simulink model "Simulink_Program_DCFC_Normal"  (R2023b)
settings: Solver=VariableStepAuto  StartTime=0.0  StopTime=1  RelTol=1e-3
libraries: fl_lib x12, nesl_utility x10, ee_lib x7
settings Model: Creator=romul  LastModifiedBy=OWNER

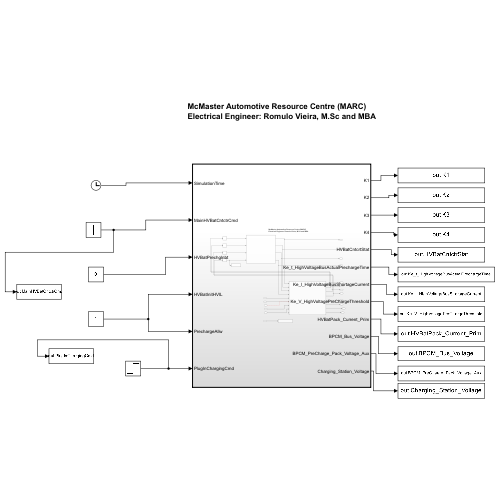
[thumbnail: Simulink's stored preview of the top-level diagram]
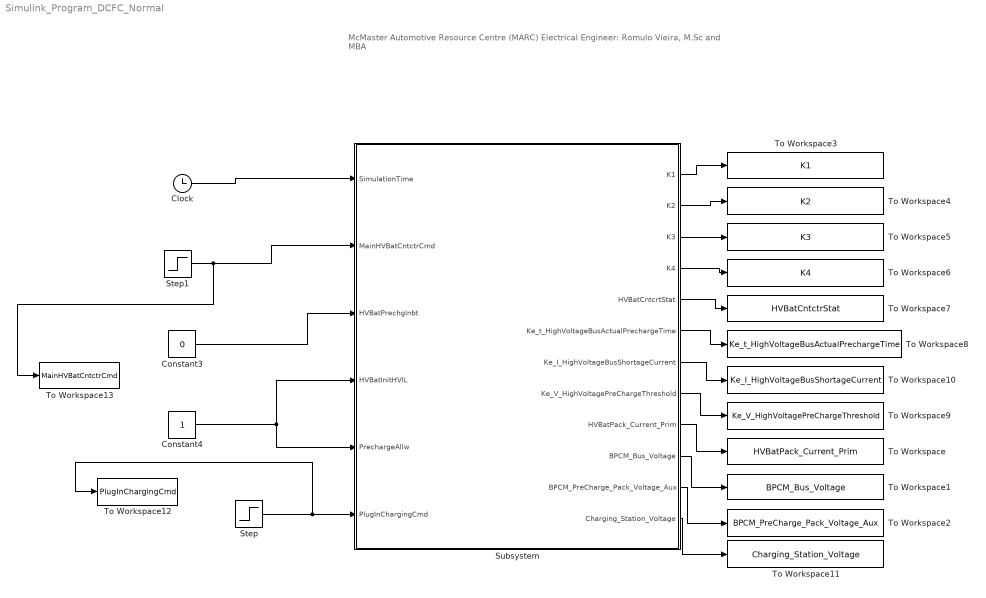
== system Simulink_Program_DCFC_Normal ==
  note: McMaster Automotive Resource Centre (MARC)
      | Electrical Engineer: Romulo Vieira, M.Sc and MBA
  Clock : Clock
  Constant3 : Constant  Value=0
  Constant4 : Constant
  Step : Step  Time=0.5  SampleTime=0.001
  Step1 : Step  Time=0.5  SampleTime=0.001
  Subsystem : Subsystem  TreatAsAtomicUnit=on
  To Workspace : ToWorkspace  VariableName=HVBatPack_Current_Prim  SampleTime=-1
  To Workspace1 : ToWorkspace  VariableName=BPCM_Bus_Voltage  SampleTime=-1
  To Workspace10 : ToWorkspace  VariableName=Ke_I_HighVoltageBusShortageCurrent  SampleTime=-1
  To Workspace11 : ToWorkspace  VariableName=Charging_Station_Voltage  SampleTime=-1
  To Workspace12 : ToWorkspace  VariableName=PlugInChargingCmd  SaveFormat=Timeseries  SampleTime=-1
  To Workspace13 : ToWorkspace  VariableName=MainHVBatCntctrCmd  SaveFormat=Timeseries  SampleTime=-1
  To Workspace2 : ToWorkspace  VariableName=BPCM_PreCharge_Pack_Voltage_Aux  SampleTime=-1
  To Workspace3 : ToWorkspace  VariableName=K1  SampleTime=-1
  To Workspace4 : ToWorkspace  VariableName=K2  SampleTime=-1
  To Workspace5 : ToWorkspace  VariableName=K3  SampleTime=-1
  To Workspace6 : ToWorkspace  VariableName=K4  SampleTime=-1
  To Workspace7 : ToWorkspace  VariableName=HVBatCntctrStat  SampleTime=-1
  To Workspace8 : ToWorkspace  VariableName=Ke_t_HighVoltageBusActualPrechargeTime  SampleTime=-1
  To Workspace9 : ToWorkspace  VariableName=Ke_V_HighVoltagePreChargeThreshold  SampleTime=-1
  wires:
  Subsystem/1(K1) -> To Workspace3/1
  Subsystem/2(K2) -> To Workspace4/1
  Subsystem/3(K3) -> To Workspace5/1
  Subsystem/4(K4) -> To Workspace6/1
  Subsystem/5(HVBatCntcrtStat) -> To Workspace7/1
  Subsystem/6(Ke_t_HighVoltageBusActualPrechargeTime) -> To Workspace8/1
  Subsystem/7(Ke_I_HighVoltageBusShortageCurrent) -> To Workspace10/1
  Clock/1 -> Subsystem/1(SimulationTime)
  Step1/1 -> To Workspace13/1, Subsystem/2(MainHVBatCntctrCmd)
  Constant3/1 -> Subsystem/3(HVBatPrechgInbt)
  Constant4/1 -> Subsystem/5(PrechargeAllw), Subsystem/4(HVBatInitHVIL)
  Subsystem/10(BPCM_Bus_Voltage) -> To Workspace1/1
  Subsystem/9(HVBatPack_Current_Prim) -> To Workspace/1
  Subsystem/11(BPCM_PreCharge_Pack_Voltage_Aux) -> To Workspace2/1
  Subsystem/8(Ke_V_HighVoltagePreChargeThreshold) -> To Workspace9/1
  Subsystem/12(Charging_Station_Voltage) -> To Workspace11/1
  Step/1 -> To Workspace12/1, Subsystem/6(PlugInChargingCmd)

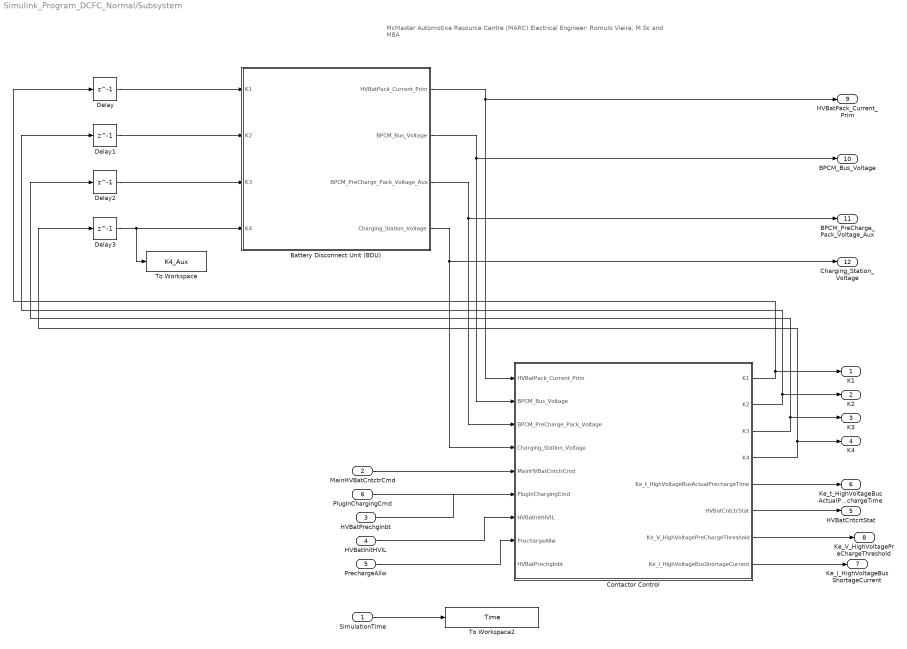
== system Simulink_Program_DCFC_Normal/Subsystem ==
  note: McMaster Automotive Resource Centre (MARC)
      | Electrical Engineer: Romulo Vieira, M.Sc and MBA
  SimulationTime : Inport
  MainHVBatCntctrCmd : Inport  Port=2
  HVBatPrechgInbt : Inport  Port=3
  HVBatInitHVIL : Inport  Port=4
  PrechargeAllw : Inport  Port=5
  PlugInChargingCmd : Inport  Port=6
  Battery Disconnect Unit (BDU) : Subsystem  TreatAsAtomicUnit=on
  Contactor Control : Subsystem  TreatAsAtomicUnit=on  SystemSampleTime=0.001
  Delay{,1..3} (4 alike) : Delay  DelayLength=1
  To Workspace : ToWorkspace  VariableName=K4_Aux  SaveFormat=Timeseries  SampleTime=-1
  To Workspace2 : ToWorkspace  VariableName=Time  SampleTime=0.001
  K1 : Outport
  K2 : Outport  Port=2
  K3 : Outport  Port=3
  K4 : Outport  Port=4
  HVBatCntcrtStat : Outport  Port=5
  Ke_t_HighVoltageBusActualPrechargeTime : Outport  Port=6
  Ke_I_HighVoltageBusShortageCurrent : Outport  Port=7
  Ke_V_HighVoltagePreChargeThreshold : Outport  Port=8
  HVBatPack_Current_Prim : Outport  Port=9
  BPCM_Bus_Voltage : Outport  Port=10
  BPCM_PreCharge_Pack_Voltage_Aux : Outport  Port=11
  Charging_Station_Voltage : Outport  Port=12
  wires:
  Battery Disconnect Unit (BDU)/1(HVBatPack_Current_Prim) -> Contactor Control/1(HVBatPack_Current_Prim), HVBatPack_Current_Prim/1
  Battery Disconnect Unit (BDU)/2(BPCM_Bus_Voltage) -> Contactor Control/2(BPCM_Bus_Voltage), BPCM_Bus_Voltage/1
  MainHVBatCntctrCmd/1 -> Contactor Control/5(MainHVBatCntctrCmd)
  HVBatPrechgInbt/1 -> ?
  HVBatInitHVIL/1 -> Contactor Control/7(HVBatInitHVIL)
  PrechargeAllw/1 -> Contactor Control/8(PrechargeAllw)
  Contactor Control/1(K1) -> K1/1, Delay/1
  Contactor Control/2(K2) -> K2/1, Delay1/1
  Contactor Control/3(K3) -> K3/1, Delay2/1
  Contactor Control/4(K4) -> K4/1, Delay3/1
  Contactor Control/6(HVBatCntctrStat) -> HVBatCntcrtStat/1
  Contactor Control/5(Ke_t_HighVoltageBusActualPrechargeTime) -> Ke_t_HighVoltageBusActualPrechargeTime/1
  Contactor Control/8(Ke_I_HighVoltageBusShortageCurrent) -> Ke_I_HighVoltageBusShortageCurrent/1
  Contactor Control/7(Ke_V_HighVoltagePreChargeThreshold) -> Ke_V_HighVoltagePreChargeThreshold/1
  Battery Disconnect Unit (BDU)/3(BPCM_PreCharge_Pack_Voltage_Aux) -> BPCM_PreCharge_Pack_Voltage_Aux/1, Contactor Control/3(BPCM_PreCharge_Pack_Voltage)
  Delay/1 -> Battery Disconnect Unit (BDU)/1(K1)
  Delay1/1 -> Battery Disconnect Unit (BDU)/2(K2)
  Delay2/1 -> Battery Disconnect Unit (BDU)/3(K3)
  Delay3/1 -> To Workspace/1, Battery Disconnect Unit (BDU)/4(K4)
  SimulationTime/1 -> To Workspace2/1
  Battery Disconnect Unit (BDU)/4(Charging_Station_Voltage) -> Charging_Station_Voltage/1, Contactor Control/4(Charging_Station_Voltage)
  PlugInChargingCmd/1 -> Contactor Control/6(PlugInChargingCmd)

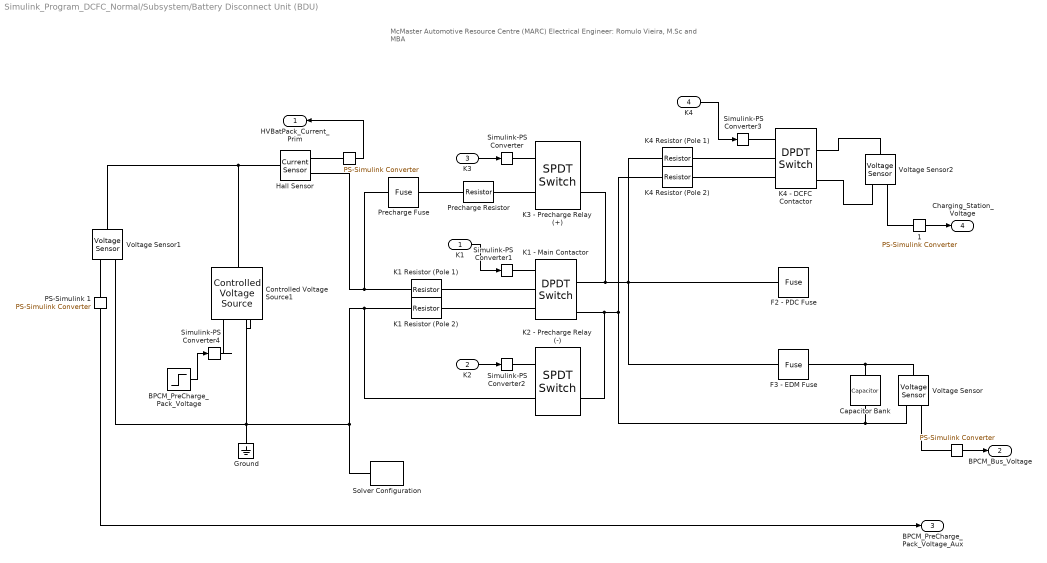
== system Simulink_Program_DCFC_Normal/Subsystem/Battery Disconnect Unit (BDU) ==
  note: McMaster Automotive Resource Centre (MARC)
      | Electrical Engineer: Romulo Vieira, M.Sc and MBA
  K1 : Inport
  K2 : Inport  Port=2
  K3 : Inport  Port=3
  K4 : Inport  Port=4
  "   " : nesl_utility/PS-Simulink Converter  PhysicalDomain=network_engine_domain  SubClassName=ps_output  LeftPortType=input  RightPortType=output  PseudoPeriodic=off  Frequencies=[]  VectorFormat=inherit  Unit=inherit  AffineConversion=off
  " " : nesl_utility/PS-Simulink Converter  PhysicalDomain=network_engine_domain  SubClassName=ps_output  LeftPortType=input  RightPortType=output  PseudoPeriodic=off  Frequencies=[]  VectorFormat=inherit  Unit=inherit  AffineConversion=off
  " 1" : nesl_utility/PS-Simulink Converter  PhysicalDomain=network_engine_domain  SubClassName=ps_output  LeftPortType=input  RightPortType=output  PseudoPeriodic=off  Frequencies=[]  VectorFormat=inherit  Unit=inherit  AffineConversion=off
  BPCM_PreCharge_Pack_Voltage : Step  Time=0  After=450  SampleTime=0.001
  Capacitor Bank : fl_lib/Electrical/Electrical Elements/Capacitor  c=750e-6 F  r=1e-6 Ohm  g=0 1/Ohm  i_specify=off  i_priority=None  i=0 A  i_nominal_specify=off  i_nominal_unit=A  i_nominal_value=1  v_specify=off  v_priority=None  v=0 V  v_nominal_specify=off  v_nominal_unit=V  v_nominal_value=1  vc_specify=on  vc_priority=High  vc=0 V  vc_nominal_specify=off  vc_nominal_unit=V  vc_nominal_value=1
  Controlled Voltage Source1 : fl_lib/Electrical/Electrical Sources/Controlled Voltage Source
  F2 - PDC Fuse : ee_lib/Switches & Breakers/Fuse  prm=1  I_rated=125 A  melt_margin=1  T_fuse=0 s  I2t=1 A^2*s  I_vec=[1.9, 2, 2.5, 30] A  t_vec=[10000, 1, .3, .001] s  R_closed=0.01 Ohm  G_open=1e-8 1/Ohm  exposemeasurement=ee.enum.exposemeasurement.hidden
      settings: InternalSimscapePortConfiguration="{\"Bottom\":[],\"Left\":[{\"id\":\"p\",\"label\":\"\",\"type\":\"foundation.electrical.electrical\"}],\"Right\":[{\"id\":\"n\",\"label\":\"\",\"type\":\"foundation.electrical.electrical\"}],\"Top\":[]}"
  F3 - EDM Fuse : ee_lib/Switches & Breakers/Fuse  prm=1  I_rated=600 A  melt_margin=1  T_fuse=0 s  I2t=1 A^2*s  I_vec=[1.9, 2, 2.5, 30] A  t_vec=[10000, 1, .3, .001] s  R_closed=0.01 Ohm  G_open=1e-8 1/Ohm  exposemeasurement=ee.enum.exposemeasurement.hidden
      settings: InternalSimscapePortConfiguration="{\"Bottom\":[],\"Left\":[{\"id\":\"p\",\"label\":\"\",\"type\":\"foundation.electrical.electrical\"}],\"Right\":[{\"id\":\"n\",\"label\":\"\",\"type\":\"foundation.electrical.electrical\"}],\"Top\":[]}"
  Ground : fl_lib/Electrical/Electrical Elements/Electrical Reference
  Hall Sensor : fl_lib/Electrical/Electrical Sensors/Current Sensor
  K1 - Main Contactor : ee_lib/Switches & Breakers/DPDT Switch  R_closed=0.01 Ohm  G_open=1e-6 S  Threshold=0.5 V  Width=0 V  model_dynamics=0  t_on=1e-3 s  t_off=1e-3 s  initial_vT=0 V
      settings: InternalSimscapePortConfiguration="{\"Bottom\":[],\"Left\":[{\"id\":\"vT\",\"label\":\"vT\",\"type\":\"input\"},{\"id\":\"p1\",\"label\":\"\",\"type\":\"foundation.electrical.electrical\"},{\"id\":\"p2\",\"label\":\"\",\"type\":\"foundation.electrical.electrical\"}],\"Right\":[{\"id\":\"n11\",\"label\":\"\",\"type\":\"foundation.electrical.electrical\"},{\"id\":\"n12\",\"label\":\"\",\"type\":\"foundation.electrical.electrical\"},{\"id\":\"n21\",\"label\":\"\",\"type\":\"foundation.electrical.electrical\"},{\"id\":\"n22\",\"label\":\"\",\"type\":\"foundation.electrical.electrical\"}],\"Top\":[]}"
  K1 Resistor (Pole 1) : fl_lib/Electrical/Electrical Elements/Resistor  R=0.0003 Ohm  i_specify=off  i_priority=None  i=0 A  i_nominal_specify=off  i_nominal_unit=A  i_nominal_value=1  v_specify=off  v_priority=None  v=0 V  v_nominal_specify=off  v_nominal_unit=V  v_nominal_value=1
  K1 Resistor (Pole 2) : fl_lib/Electrical/Electrical Elements/Resistor  R=0.0003 Ohm  i_specify=off  i_priority=None  i=0 A  i_nominal_specify=off  i_nominal_unit=A  i_nominal_value=1  v_specify=off  v_priority=None  v=0 V  v_nominal_specify=off  v_nominal_unit=V  v_nominal_value=1
  K2 - Precharge Relay (-) : ee_lib/Switches & Breakers/SPDT Switch  R_closed=0.01 Ohm  G_open=1e-6 S  Threshold=0.5 V  Width=0 V  model_dynamics=0  t_on=1e-3 s  t_off=1e-3 s  initial_vT=0 V
  K3 - Precharge Relay (+) : ee_lib/Switches & Breakers/SPDT Switch  R_closed=0.01 Ohm  G_open=1e-6 S  Threshold=0.5 V  Width=0 V  model_dynamics=0  t_on=1e-3 s  t_off=1e-3 s  initial_vT=0 V
  K4 - DCFC Contactor : ee_lib/Switches & Breakers/DPDT Switch  R_closed=0.01 Ohm  G_open=1e-6 S  Threshold=0.5 V  Width=0 V  model_dynamics=0  t_on=1e-3 s  t_off=1e-3 s  initial_vT=0 V
      settings: InternalSimscapePortConfiguration="{\"Bottom\":[],\"Left\":[{\"id\":\"vT\",\"label\":\"vT\",\"type\":\"input\"},{\"id\":\"p1\",\"label\":\"\",\"type\":\"foundation.electrical.electrical\"},{\"id\":\"p2\",\"label\":\"\",\"type\":\"foundation.electrical.electrical\"}],\"Right\":[{\"id\":\"n11\",\"label\":\"\",\"type\":\"foundation.electrical.electrical\"},{\"id\":\"n12\",\"label\":\"\",\"type\":\"foundation.electrical.electrical\"},{\"id\":\"n21\",\"label\":\"\",\"type\":\"foundation.electrical.electrical\"},{\"id\":\"n22\",\"label\":\"\",\"type\":\"foundation.electrical.electrical\"}],\"Top\":[]}"
  K4 Resistor (Pole 1) : fl_lib/Electrical/Electrical Elements/Resistor  R=0.0003 Ohm  i_specify=off  i_priority=None  i=0 A  i_nominal_specify=off  i_nominal_unit=A  i_nominal_value=1  v_specify=off  v_priority=None  v=0 V  v_nominal_specify=off  v_nominal_unit=V  v_nominal_value=1
  K4 Resistor (Pole 2) : fl_lib/Electrical/Electrical Elements/Resistor  R=0.0003 Ohm  i_specify=off  i_priority=None  i=0 A  i_nominal_specify=off  i_nominal_unit=A  i_nominal_value=1  v_specify=off  v_priority=None  v=0 V  v_nominal_specify=off  v_nominal_unit=V  v_nominal_value=1
  PS-Simulink 1 : nesl_utility/PS-Simulink Converter  PhysicalDomain=network_engine_domain  SubClassName=ps_output  LeftPortType=input  RightPortType=output  PseudoPeriodic=off  Frequencies=[]  VectorFormat=inherit  Unit=inherit  AffineConversion=off
  Precharge Fuse : ee_lib/Switches & Breakers/Fuse  prm=1  I_rated=600 A  melt_margin=1  T_fuse=0 s  I2t=1 A^2*s  I_vec=[1.9, 2, 2.5, 30] A  t_vec=[10000, 1, .3, .001] s  R_closed=0.01 Ohm  G_open=1e-8 1/Ohm  exposemeasurement=ee.enum.exposemeasurement.hidden
      settings: InternalSimscapePortConfiguration="{\"Bottom\":[],\"Left\":[{\"id\":\"p\",\"label\":\"\",\"type\":\"foundation.electrical.electrical\"}],\"Right\":[{\"id\":\"n\",\"label\":\"\",\"type\":\"foundation.electrical.electrical\"}],\"Top\":[]}"
  Precharge Resistor : fl_lib/Electrical/Electrical Elements/Resistor  R=25 Ohm  i_specify=off  i_priority=None  i=0 A  i_nominal_specify=off  i_nominal_unit=A  i_nominal_value=1  v_specify=off  v_priority=None  v=0 V  v_nominal_specify=off  v_nominal_unit=V  v_nominal_value=1
  Simulink-PS Converter{,1..3} (4 alike) : nesl_utility/Simulink-PS Converter  PhysicalDomain=network_engine_domain  SubClassName=ps_input  LeftPortType=input  RightPortType=output  PseudoPeriodic=off  Frequencies=[]  NoiseDistribution=none  NoiseParameters=[]  Unit=1  AffineConversion=off  FilteringAndDerivatives=provide  SimscapeFilterOrder=1  InputFilterTimeConstant=0.001  UdotUserProvided=0
  Simulink-PS Converter4 : nesl_utility/Simulink-PS Converter  PhysicalDomain=network_engine_domain  SubClassName=ps_input  LeftPortType=input  RightPortType=output  PseudoPeriodic=off  Frequencies=[]  NoiseDistribution=none  NoiseParameters=[]  Unit=1  AffineConversion=off  FilteringAndDerivatives=filter  SimscapeFilterOrder=1  InputFilterTimeConstant=0.0000001  UdotUserProvided=0
  Solver Configuration : nesl_utility/Solver Configuration  PhysicalDomain=network_engine_domain  SubClassName=solver  LeftPortType=input  RightPortType=generic  Tones=[]  Harmonics=[]  SimulateNoise=off  Profile=off  UseLocalSampling=off  EnableSwitchedLinearOptims=on  FrequencyDomain=off  UseCCode=off  RelTol=0.001  AbsTol=0.001  MinStep=1e-09  ToWorkspace=off  RevertToSquareIcSolve=off  NumHomotopyIterations=100  PhasorMode=off  PhasorModeNumHarmonics=1  ConsistencySolver=NEWTON_XTOL_AFTER_FTOL  IndexReductionMethod=DerivativeReplacement  DoDC=off  ResidualTolerance=1e-09  ConsistencyTolSource=GLOBAL  ConsistencyAbsTol=0.001  ConsistencyRelTol=0.001  ConsistencyTolFactor=0.001  UseLocalSolver=off  LocalSolverChoice=NE_BACKWARD_EULER_ADVANCER  ResolveIndetEquations=on  FunctionEvalNumThread=1  LocalSolverSampleTime=0.001  DoFixedCost=off  MaxNonlinIter=3  MaxModeIter=2  ComputeImpulses=off  ImpulseIterations=2  LinearAlgebra=auto  LinearAlgebraNumThread=0  EquationFormulation=NE_TIME_EF  DelaysMemoryBudget=1024  AutomaticFiltering=on  FilteringTimeConstant=0.001  PartitionStorageMethod=AS_NEEDED  PartitionMemoryBudget=1024  PartitionMethod=ROBUST  MultibodyUseLocalSolver=off  MultibodyLocalSolverChoice=ODE1  MultibodyLocalSolverSampleTime=0.001
  Voltage Sensor : fl_lib/Electrical/Electrical Sensors/Voltage Sensor
  Voltage Sensor1 : fl_lib/Electrical/Electrical Sensors/Voltage Sensor
  Voltage Sensor2 : fl_lib/Electrical/Electrical Sensors/Voltage Sensor
  HVBatPack_Current_Prim : Outport
  BPCM_Bus_Voltage : Outport  Port=2
  BPCM_PreCharge_Pack_Voltage_Aux : Outport  Port=3
  Charging_Station_Voltage : Outport  Port=4
  wires:
  K4/1 -> Simulink-PS Converter3/1
  K3/1 -> Simulink-PS Converter/1
  "   "/1 -> HVBatPack_Current_Prim/1
  K1/1 -> Simulink-PS Converter1/1
  K2/1 -> Simulink-PS Converter2/1
  BPCM_PreCharge_Pack_Voltage/1 -> Simulink-PS Converter4/1
  " "/1 -> BPCM_Bus_Voltage/1
  PS-Simulink 1/1 -> BPCM_PreCharge_Pack_Voltage_Aux/1
  " 1"/1 -> Charging_Station_Voltage/1
  connections:
  K1 Resistor (Pole 2)/LConn1 -- K1 - Main Contactor/LConn3
  Capacitor Bank/LConn1 -- Voltage Sensor/LConn1 -- F3 - EDM Fuse/LConn1
  K2 - Precharge Relay (-)/RConn2 -- K1 - Main Contactor/RConn4 -- Voltage Sensor/RConn2 -- Capacitor Bank/RConn1 -- K4 Resistor (Pole 2)/RConn1
  Hall Sensor/RConn2 -- Precharge Fuse/LConn1 -- K1 Resistor (Pole 1)/RConn1
  K3 - Precharge Relay (+)/RConn2 -- K4 Resistor (Pole 1)/RConn1 -- F2 - PDC Fuse/RConn1 -- F3 - EDM Fuse/RConn1 -- K1 - Main Contactor/RConn2
  Precharge Resistor/LConn1 -- K3 - Precharge Relay (+)/LConn2
  Simulink-PS Converter2/RConn1 -- K2 - Precharge Relay (-)/LConn1
  Precharge Resistor/RConn1 -- Precharge Fuse/RConn1
  Simulink-PS Converter1/RConn1 -- K1 - Main Contactor/LConn1
  Controlled Voltage Source1/LConn1 -- Hall Sensor/LConn1 -- Voltage Sensor1/LConn1
  Simulink-PS Converter/RConn1 -- K3 - Precharge Relay (+)/LConn1
  Voltage Sensor/RConn1 -- " "/LConn1
  K4 - DCFC Contactor/LConn1 -- Simulink-PS Converter3/RConn1
  "   "/LConn1 -- Hall Sensor/RConn1
  Simulink-PS Converter4/RConn1 -- Controlled Voltage Source1/RConn1
  Voltage Sensor1/RConn1 -- PS-Simulink 1/LConn1
  K1 Resistor (Pole 1)/LConn1 -- K1 - Main Contactor/LConn2
  Solver Configuration/RConn1 -- Ground/LConn1 -- Voltage Sensor1/RConn2 -- Controlled Voltage Source1/RConn2 -- K2 - Precharge Relay (-)/LConn2 -- K1 Resistor (Pole 2)/RConn1
  K4 - DCFC Contactor/LConn2 -- K4 Resistor (Pole 1)/LConn1
  K4 Resistor (Pole 2)/LConn1 -- K4 - DCFC Contactor/LConn3
  K4 - DCFC Contactor/RConn2 -- Voltage Sensor2/LConn1
  K4 - DCFC Contactor/RConn4 -- Voltage Sensor2/RConn2
  " 1"/LConn1 -- Voltage Sensor2/RConn1

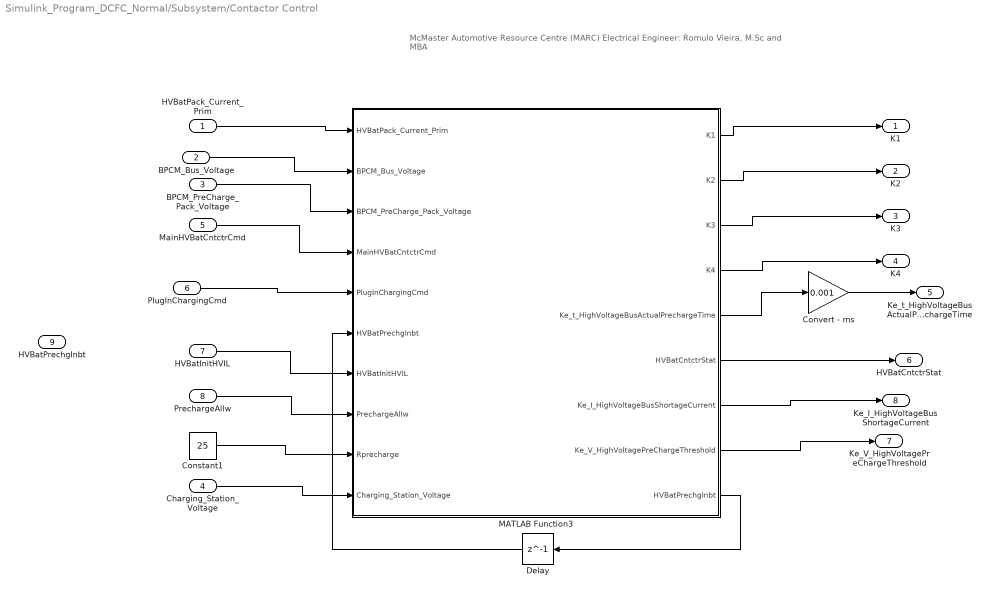
== system Simulink_Program_DCFC_Normal/Subsystem/Contactor Control ==
  note: McMaster Automotive Resource Centre (MARC)
      | Electrical Engineer: Romulo Vieira, M.Sc and MBA
  HVBatPack_Current_Prim : Inport
  BPCM_Bus_Voltage : Inport  Port=2
  BPCM_PreCharge_Pack_Voltage : Inport  Port=3
  Charging_Station_Voltage : Inport  Port=4
  MainHVBatCntctrCmd : Inport  Port=5
  PlugInChargingCmd : Inport  Port=6
  HVBatInitHVIL : Inport  Port=7
  PrechargeAllw : Inport  Port=8
  HVBatPrechgInbt : Inport  Port=9
  Constant1 : Constant  Value=25
  Convert - ms : Gain  Gain=0.001
  Delay : Delay  DelayLength=1
  MATLAB Function3 : MATLAB Function  SystemSampleTime=0.001
  K1 : Outport
  K2 : Outport  Port=2
  K3 : Outport  Port=3
  K4 : Outport  Port=4
  Ke_t_HighVoltageBusActualPrechargeTime : Outport  Port=5
  HVBatCntctrStat : Outport  Port=6
  Ke_V_HighVoltagePreChargeThreshold : Outport  Port=7
  Ke_I_HighVoltageBusShortageCurrent : Outport  Port=8
  wires:
  Constant1/1 -> MATLAB Function3/9(Rprecharge)
  HVBatInitHVIL/1 -> MATLAB Function3/7(HVBatInitHVIL)
  MainHVBatCntctrCmd/1 -> MATLAB Function3/4(MainHVBatCntctrCmd)
  HVBatPack_Current_Prim/1 -> MATLAB Function3/1(HVBatPack_Current_Prim)
  PrechargeAllw/1 -> MATLAB Function3/8(PrechargeAllw)
  MATLAB Function3/1(K1) -> K1/1
  BPCM_PreCharge_Pack_Voltage/1 -> MATLAB Function3/3(BPCM_PreCharge_Pack_Voltage)
  Charging_Station_Voltage/1 -> MATLAB Function3/10(Charging_Station_Voltage)
  MATLAB Function3/2(K2) -> K2/1
  MATLAB Function3/3(K3) -> K3/1
  MATLAB Function3/4(K4) -> K4/1
  MATLAB Function3/6(HVBatCntctrStat) -> HVBatCntctrStat/1
  MATLAB Function3/7(Ke_I_HighVoltageBusShortageCurrent) -> Ke_I_HighVoltageBusShortageCurrent/1
  MATLAB Function3/9(HVBatPrechgInbt) -> Delay/1
  Delay/1 -> MATLAB Function3/6("HVBatPrechgInbt ")
  BPCM_Bus_Voltage/1 -> MATLAB Function3/2(BPCM_Bus_Voltage)
  MATLAB Function3/8(Ke_V_HighVoltagePreChargeThreshold) -> Ke_V_HighVoltagePreChargeThreshold/1
  Convert - ms/1 -> Ke_t_HighVoltageBusActualPrechargeTime/1
  MATLAB Function3/5(Ke_t_HighVoltageBusActualPrechargeTime) -> Convert - ms/1
  PlugInChargingCmd/1 -> MATLAB Function3/5(PlugInChargingCmd)

== matlab function Simulink_Program_DCFC_Normal/Subsystem/Contactor Control/MATLAB Function3 ==
  data: HVBatPack_Current_Prim input; BPCM_Bus_Voltage input; BPCM_PreCharge_Pack_Voltage input; MainHVBatCntctrCmd input; PlugInChargingCmd input; K1 output; HVBatPrechgInbt input; HVBatInitHVIL input; PrechargeAllw input; K2 output; K3 output; K4 output; Ke_t_HighVoltageBusActualPrechargeTime output; HVBatCntctrStat output; Ke_I_HighVoltageBusShortageCurrent output; Ke_V_HighVoltagePreChargeThreshold output; Rprecharge input; HVBatPrechgInbt output; Charging_Station_Voltage input
function [K1, K2, K3, K4, Ke_t_HighVoltageBusActualPrechargeTime, HVBatCntctrStat, Ke_I_HighVoltageBusShortageCurrent, Ke_V_HighVoltagePreChargeThreshold, HVBatPrechgInbt] = ...
    prechargeSequencerNoClock(HVBatPack_Current_Prim, BPCM_Bus_Voltage, ...
    BPCM_PreCharge_Pack_Voltage, MainHVBatCntctrCmd, PlugInChargingCmd, HVBatPrechgInbt, HVBatInitHVIL, PrechargeAllw, Rprecharge, Charging_Station_Voltage)

%-----------------------------------------------------------
% McMaster Automotive Resource Centre (MARC)
% Electrical Engineer: Romulo Vieira, M.Sc and MBA - PhD Candidate
%-----------------------------------------------------------
% Purpose: Manage precharge relay and contactor sequence with retry + inhibit logic
%-----------------------------------------------------------

% HVBatCntctrStat Mapping:
% 0 – Idle/Waiting
% 1 – Precharge Active
% 2 – Precharge Complete (Main contactors closed)
% 3 - DCFC Charging
% 4 – Precharge Failed
% 5 – Inhibit State (cooldown after failure)
% 6 – Contactor Control Shorted (high or low)
% 7 - SNA (Signal Not Available)

% --- Constants ---
Unset_VbusTargetHitIdx             = -1;   % Flag indicating Vbus threshold not yet hit
Min_Samples                        = 0;    % Minimum number of samples where relays and contactor are both active

% Internal Configuration Parameters
Ke_t_PrechargeFailCoolTime             = 3000;   % Cooldown time after one single failed attempt [ms]
Ke_t_ExtraPrechargeFailCoolPenaltyTime = 2000;   % Additional cooldown after two multiple failures [ms]
Ke_t_PrechargeFailMaxPenalty           = 10000;  % Maximum time threshold before enabling precharge inhibit state
Ke_t_BPCM_Precharge_Fail_Penalty_Time  = 15000;  % Hard inhibit time if failures persist [ms]
Ke_I_HighVoltageBusShortageCurrentMin  = 10.8;   % Minimum expected precharge current [A]
Ke_V_HighVoltagePreChargeThreshold     = 0.993 * BPCM_PreCharge_Pack_Voltage;  % Target voltage threshold
Ke_t_HighVoltageBusPrechargeTime  = 100;    % Maximum allowable time for precharging [ms]

% --- Persistent Variables ---
persistent I_buffer idx HVBatCntctrStat_Aux VbusTargetHitIdx ...
    t_counter last_PrechargeAllw Prchrgpnltytimer PrechargeFailCount

if isempty(I_buffer)
    I_buffer               = zeros(Ke_t_HighVoltageBusPrechargeTime,1);
    idx                    = 1;
    HVBatCntctrStat_Aux    = 0;
    VbusTargetHitIdx       = Unset_VbusTargetHitIdx;
    t_counter              = 0;
    last_PrechargeAllw     = 0;
    Prchrgpnltytimer       = 0;
    PrechargeFailCount     = 0; % Represented by k_fail in the flowchart
end

% --- Default Outputs ---
K1 = 0; K2 = 0; K3 = 0; K4 = 0;
HVBatCntctrStat = HVBatCntctrStat_Aux;
Ke_t_HighVoltageBusActualPrechargeTime = 0;
Ke_I_HighVoltageBusShortageCurrent = 0;

% --- Immediate cooldown/inhibit override ---
if Prchrgpnltytimer > 0 && HVBatCntctrStat_Aux ~= 5
    HVBatCntctrStat_Aux = 5;
end

% --- State Machine ---
switch HVBatCntctrStat_Aux
    case 0 % OPEN STATE
        % Set the Battery Contactor States
        K1 = 0; K2 = 0; K3 = 0; K4 = 0;
        % Check Initial conditions
        if PlugInChargingCmd == 1 && MainHVBatCntctrCmd == 1 && HVBatPrechgInbt == 0 && HVBatInitHVIL == 1 && PrechargeAllw == 1
            HVBatCntctrStat_Aux = 3; % DCFC CHARGING
        end
        if PlugInChargingCmd == 0 && MainHVBatCntctrCmd == 1 && HVBatPrechgInbt == 0 && HVBatInitHVIL == 1  && PrechargeAllw == 1
            I_buffer(:) = 0;
            idx = 1;
            VbusTargetHitIdx = Unset_VbusTargetHitIdx;
            t_counter = 0;
            HVBatCntctrStat_Aux = 1;
        end

    case 1  % PRECHARGING STATE
        % Move to DCFC charging state
        if PlugInChargingCmd == 1
            HVBatCntctrStat_Aux = 3; % DCFC CHARGING
        end

        % Abort if initial conditions are no longer valid
        if MainHVBatCntctrCmd ~= 1 || HVBatPrechgInbt ~= 0 || HVBatInitHVIL ~= 1 || PrechargeAllw ~= 1
            HVBatCntctrStat_Aux = 0;
            return;
        end

        % Set precharge relays ON
        K1 = 0; K2 = 1; K3 = 1; K4 = 0;

        % Record current
        if t_counter == 0
            I_buffer(idx) = BPCM_PreCharge_Pack_Voltage / Rprecharge;
        else
            I_buffer(idx) = HVBatPack_Current_Prim;
        end
        Ke_I_HighVoltageBusShortageCurrent = max(I_buffer);

        % Voltage target check
        if VbusTargetHitIdx == Unset_VbusTargetHitIdx && BPCM_Bus_Voltage >= Ke_V_HighVoltagePreChargeThreshold
            VbusTargetHitIdx = t_counter + 1;
        end

        % Time since start or since target hit
        if VbusTargetHitIdx ~= Unset_VbusTargetHitIdx
            delta_samples = VbusTargetHitIdx;
        else
            delta_samples = t_counter;
        end

        % SUCCESS - PRECHARGE CONDITIONS ARE MET
        if t_counter < Ke_t_HighVoltageBusPrechargeTime && ... 
                VbusTargetHitIdx ~= Unset_VbusTargetHitIdx && delta_samples < Ke_t_HighVoltageBusPrechargeTime && Ke_I_HighVoltageBusShortageCurrent >= Ke_I_HighVoltageBusShortageCurrentMin
            
            % Set the next Battery Contactor Status
            HVBatCntctrStat_Aux = 2;
            % Set the Battery Contactor States
            K1 = 1; K2 = 0; K3 = 0; K4 = 0;

            PrechargeFailCount = 0;
            Prchrgpnltytimer = 0;

        % FAILURE - PRECHARGE CONDITIONS ARE NOT MET
        elseif t_counter == Ke_t_HighVoltageBusPrechargeTime && ...
               (VbusTargetHitIdx == Unset_VbusTargetHitIdx || delta_samples == Ke_t_HighVoltageBusPrechargeTime || Ke_I_HighVoltageBusShortageCurrent < Ke_I_HighVoltageBusShortageCurrentMin)

            % Set the Battery Contactor States
            K1 = 0; K2 = 0; K3 = 0; K4 = 0;
           % Set the Battery Contactor Status
            HVBatCntctrStat_Aux = 4;

            % Update the total cooling time before re-attempt
            PrechargeFailCount = PrechargeFailCount + 1;
            Prchrgpnltytimer = Prchrgpnltytimer + Ke_t_PrechargeFailCoolTime;

            if PrechargeFailCount >= 2
                Prchrgpnltytimer = Prchrgpnltytimer + Ke_t_ExtraPrechargeFailCoolPenaltyTime;
            end

            % Check PRECHARGE INHIBIT CONDITIONS:
            if Prchrgpnltytimer > Ke_t_PrechargeFailMaxPenalty % Include the here || (HVBatPrechargeTemp > 60) 
                % Set the next Battery Contactor Status
                HVBatCntctrStat_Aux = 5;
                HVBatPrechgInbt = 1;
                Prchrgpnltytimer = Ke_t_BPCM_Precharge_Fail_Penalty_Time;
            end

        end

        % Update counters
        t_counter = t_counter + 1;
        idx = idx + 1;
        if idx > Ke_t_HighVoltageBusPrechargeTime, idx = 1; end

    case 2  % PRECHARGE COMPLETE OR CLOSED
        % Set the Battery Contactor States
        K1 = 1; K2 = 0; K3 = 0; K4 = 0;

        if PlugInChargingCmd == 1
            HVBatCntctrStat_Aux = 3; % DCFC CHARGING
        end

        if last_PrechargeAllw == 0 && PrechargeAllw == 1
            HVBatCntctrStat_Aux = 0;
            I_buffer(:) = 0;
            idx = 1;
            VbusTargetHitIdx = Unset_VbusTargetHitIdx;
            t_counter = 0;
        end

    case 3 % DCFC CHARGING
        % Set the Battery Contactor States
        K1 = 1; K2 = 0; K3 = 0; K4 = 1;

        if ~(MainHVBatCntctrCmd == 1 && PlugInChargingCmd == 1)
            if MainHVBatCntctrCmd == 0
                HVBatCntctrStat_Aux = 0; % OPEN
            else
                HVBatCntctrStat_Aux = 2; % CLOSED
            end
        end


    case 4  % PRECHARGE FAILED STATE
        % Set the Battery Contactor States
        K1 = 0; K2 = 0; K3 = 0; K4 = 0;
        if Prchrgpnltytimer > 0
            Prchrgpnltytimer = Prchrgpnltytimer - 1;
        else
            HVBatCntctrStat_Aux = 0;
        end

    case 5  % PRECHARGE INHIBIT STATE
        % Set the Battery Contactor States
        K1 = 0; K2 = 0; K3 = 0; K4 = 0;

        if Prchrgpnltytimer > 0
            Prchrgpnltytimer = Prchrgpnltytimer - 1;
        else
            % Cooldown finished → check if PRECHARGE INHIBIT conditions still exist
            if (Prchrgpnltytimer > Ke_t_PrechargeFailMaxPenalty) % Include the here || (HVBatPrechargeTemp > 60)
                % Inhibit condition persists → apply long penalty
                Prchrgpnltytimer = Ke_t_BPCM_Precharge_Fail_Penalty_Time;
                HVBatCntctrStat_Aux = 5;
                HVBatPrechgInbt = 1;
            else
                % PRECHARGE INHIBIT conditions cleared → ready for retry
                Prchrgpnltytimer = 0;
                HVBatPrechgInbt = 0;
                HVBatCntctrStat_Aux = 0;
            end
        end


    otherwise
        K1 = 0; K2 = 0; K3 = 0; K4 = 0;
        HVBatCntctrStat_Aux = 0;
end

% --- Final Outputs ---
HVBatCntctrStat = HVBatCntctrStat_Aux;
Ke_t_HighVoltageBusActualPrechargeTime = max(0, VbusTargetHitIdx + ...
    Min_Samples * (VbusTargetHitIdx ~= Unset_VbusTargetHitIdx));
last_PrechargeAllw = PrechargeAllw;

end





















% function [K1, K2, K3, K4, HVBatCntctrStat, Ke_I_HighVoltageBusShortageCurrent, Ke_V_HighVoltagePreChargeThreshold, HVBatPrechgInbt] = ...
%     prechargeSequencerNoClock(HVBatPack_Current_Prim, BPCM_Bus_Voltage, ...
%     BPCM_PreCharge_Pack_Voltage, MainHVBatCntctrCmd, PlugInChargingCmd, HVBatPrechgInbt, HVBatInitHVIL, PrechargeAllw, Rprecharge, Charging_Station_Voltage)
% 
% %-----------------------------------------------------------
% % McMaster Automotive Resource Centre (MARC)
% % Electrical Engineer: Romulo Vieira, M.Sc and MBA - PhD Candidate
% %-----------------------------------------------------------
% % Purpose: Manage precharge relay and contactor sequence with retry + inhibit logic
% %-----------------------------------------------------------
% 
% % HVBatCntctrStat Mapping:
% % 0 – Idle/Waiting
% % 1 – Precharge Active
% % 2 – Precharge Complete (Main contactors closed)
% % 3 - DCFC Charging
% % 4 – Precharge Failed
% % 5 – Inhibit State (cooldown after failure)
% % 6 – Contactor Control Shorted (high or low)
% % 7 - SNA (Signal Not Available)
% 
% % --- Constants ---
% Unset_VbusTargetHitIdx             = -1;   % Flag indicating Vbus threshold not yet hit
% Min_Samples                        = 0;    % Minimum number of samples where relays and contactor are both active
% 
% % Internal Configuration Parameters
% Ke_t_PrechargeFailCoolTime             = 3000;   % Cooldown time after one single failed attempt [ms]
% Ke_t_ExtraPrechargeFailCoolPenaltyTime = 2000;   % Additional cooldown after two multiple failures [ms]
% Ke_t_PrechargeFailMaxPenalty           = 10000;  % Maximum time threshold before enabling precharge inhibit state
% Ke_t_BPCM_Precharge_Fail_Penalty_Time  = 15000;  % Hard inhibit time if failures persist [ms]
% Ke_I_HighVoltageBusShortageCurrentMin  = 10.8;   % Minimum expected precharge current [A]
% Ke_V_HighVoltagePreChargeThreshold     = 0.993 * BPCM_PreCharge_Pack_Voltage;  % Target voltage threshold
% Ke_t_HighVoltageBusPrechargeTime  = 100;    % Maximum allowable time for precharging [ms]
% 
% % --- Persistent Variables ---
% persistent I_buffer idx HVBatCntctrStat_Aux VbusTargetHitIdx ...
%     t_counter last_PrechargeAllw Prchrgpnltytimer PrechargeFailCount
% 
% if isempty(I_buffer)
%     I_buffer               = zeros(Ke_t_HighVoltageBusPrechargeTime,1);
%     idx                    = 1;
%     HVBatCntctrStat_Aux    = 0;
%     VbusTargetHitIdx       = Unset_VbusTargetHitIdx;
%     t_counter              = 0;
%     last_PrechargeAllw     = 0;
%     Prchrgpnltytimer       = 0;
%     PrechargeFailCount     = 0; % Represented by k_fail in the flowchart
% end
% 
% % --- Default Outputs ---
% K1 = 0; K2 = 0; K3 = 0; K4 = 0;
% HVBatCntctrStat = HVBatCntctrStat_Aux;
% Ke_t_HighVoltageBusActualPrechargeTime = 0;
% Ke_I_HighVoltageBusShortageCurrent = 0;
% 
% % --- Immediate cooldown/inhibit override ---
% if Prchrgpnltytimer > 0 && HVBatCntctrStat_Aux ~= 5
%     HVBatCntctrStat_Aux = 5;
% end
% 
% % --- State Machine ---
% switch HVBatCntctrStat_Aux
%     case 0 % OPEN STATE
%         % Set the Battery Contactor States
%         K1 = 0; K2 = 0; K3 = 0; K4 = 0;
%         % Check Initial conditions
%         if PlugInChargingCmd == 1 && MainHVBatCntctrCmd == 1 && HVBatPrechgInbt == 0 && HVBatInitHVIL == 1 && PrechargeAllw == 1
%             HVBatCntctrStat_Aux = 3; % DCFC CHARGING
%         % if PlugInChargingCmd == 1 && MainHVBatCntctrCmd == 1 
%         %     HVBatCntctrStat_Aux = 3; % DCFC CHARGING
%         elseif MainHVBatCntctrCmd == 1 && HVBatPrechgInbt == 0 && HVBatInitHVIL == 1 && PrechargeAllw == 1  && PlugInChargingCmd == 0
%             I_buffer(:) = 0;
%             idx = 1;
%             VbusTargetHitIdx = Unset_VbusTargetHitIdx;
%             t_counter = 0;
%             HVBatCntctrStat_Aux = 1;
%         end
% 
%     case 1  % PRECHARGING STATE
%         % Move to DCFC charging state
%         if PlugInChargingCmd == 1
%             HVBatCntctrStat_Aux = 3; % DCFC CHARGING
%             return;
%         end
% 
%         % Abort if initial conditions are no longer valid
%         if MainHVBatCntctrCmd ~= 1 || HVBatPrechgInbt ~= 0 || HVBatInitHVIL ~= 1 || PrechargeAllw ~= 1
%             HVBatCntctrStat_Aux = 0;
%             return;
%         end
% 
%         % Set precharge relays ON
%         K1 = 0; K2 = 1; K3 = 1; K4 = 0;
% 
%         % Record current
%         if t_counter == 0
%             I_buffer(idx) = BPCM_PreCharge_Pack_Voltage / Rprecharge;
%         else
%             I_buffer(idx) = HVBatPack_Current_Prim;
%         end
%         Ke_I_HighVoltageBusShortageCurrent = max(I_buffer);
% 
%         % Voltage target check
%         if VbusTargetHitIdx == Unset_VbusTargetHitIdx && BPCM_Bus_Voltage >= Ke_V_HighVoltagePreChargeThreshold
%             VbusTargetHitIdx = t_counter + 1;
%         end
% 
%         % Time since start or since target hit
%         if VbusTargetHitIdx ~= Unset_VbusTargetHitIdx
%             delta_samples = VbusTargetHitIdx;
%         else
%             delta_samples = t_counter;
%         end
% 
%         % SUCCESS - PRECHARGE CONDITIONS ARE MET
%         if t_counter < Ke_t_HighVoltageBusPrechargeTime && ... 
%                 VbusTargetHitIdx ~= Unset_VbusTargetHitIdx && delta_samples < Ke_t_HighVoltageBusPrechargeTime && Ke_I_HighVoltageBusShortageCurrent >= Ke_I_HighVoltageBusShortageCurrentMin
% 
%             % Set the next Battery Contactor Status
%             HVBatCntctrStat_Aux = 2;
%             % Set the Battery Contactor States
%             K1 = 1; K2 = 0; K3 = 0; K4 = 0;
% 
%             PrechargeFailCount = 0;
%             Prchrgpnltytimer = 0;
% 
%         % FAILURE - PRECHARGE CONDITIONS ARE NOT MET
%         elseif t_counter == Ke_t_HighVoltageBusPrechargeTime && ...
%                (VbusTargetHitIdx == Unset_VbusTargetHitIdx || delta_samples == Ke_t_HighVoltageBusPrechargeTime || Ke_I_HighVoltageBusShortageCurrent < Ke_I_HighVoltageBusShortageCurrentMin)
% 
%             % Set the Battery Contactor States
%             K1 = 0; K2 = 0; K3 = 0; K4 = 0;
%            % Set the Battery Contactor Status
%             HVBatCntctrStat_Aux = 4;
% 
%             % Update the total cooling time before re-attempt
%             PrechargeFailCount = PrechargeFailCount + 1;
%             Prchrgpnltytimer = Prchrgpnltytimer + Ke_t_PrechargeFailCoolTime;
% 
%             if PrechargeFailCount >= 2
%                 Prchrgpnltytimer = Prchrgpnltytimer + Ke_t_ExtraPrechargeFailCoolPenaltyTime;
%             end
% 
%             % Check PRECHARGE INHIBIT CONDITIONS:
%             if Prchrgpnltytimer > Ke_t_PrechargeFailMaxPenalty % Include the here || (HVBatPrechargeTemp > 60) 
%                 % Set the next Battery Contactor Status
%                 HVBatCntctrStat_Aux = 5;
%                 HVBatPrechgInbt = 1;
%                 Prchrgpnltytimer = Ke_t_BPCM_Precharge_Fail_Penalty_Time;
%             end
% 
%         end
% 
%         % Update counters
%         t_counter = t_counter + 1;
%         idx = idx + 1;
%         if idx > Ke_t_HighVoltageBusPrechargeTime, idx = 1; end
% 
%     case 2  % PRECHARGE COMPLETE OR CLOSED
%         % Set the Battery Contactor States
%         K1 = 1; K2 = 0; K3 = 0; K4 = 0;
% 
%         if PlugInChargingCmd == 1
%             HVBatCntctrStat_Aux = 3; % DCFC CHARGING
%         end
% 
%         if last_PrechargeAllw == 0 && PrechargeAllw == 1
%             HVBatCntctrStat_Aux = 0;
%             I_buffer(:) = 0;
%             idx = 1;
%             VbusTargetHitIdx = Unset_VbusTargetHitIdx;
%             t_counter = 0;
%         end
% 
%         if BPCM_Bus_Voltage > 270 && MainHVBatCntctrCmd == 0
%             HVBatCntctrStat_Aux = 6; % Contactor Control Shorted
%         end
% 
% 
% 
% 
%     case 3 % DCFC CHARGING
%         % Set the Battery Contactor States
%         K1 = 1; K2 = 0; K3 = 0; K4 = 1;
% 
%         if ~(MainHVBatCntctrCmd == 1 && PlugInChargingCmd == 1)
%             if MainHVBatCntctrCmd == 0
%                 HVBatCntctrStat_Aux = 0; % OPEN
%             else
%                 HVBatCntctrStat_Aux = 2; % CLOSED
%             end
%         end
% 
%     case 4  % PRECHARGE FAILED STATE
%         % Set the Battery Contactor States
%         K1 = 0; K2 = 0; K3 = 0; K4 = 0;
% 
%         if Prchrgpnltytimer > 0
%             Prchrgpnltytimer = Prchrgpnltytimer - 1;
%         else
%             HVBatCntctrStat_Aux = 0;
%         end
% 
%     case 5  % PRECHARGE INHIBIT STATE
%         % Set the Battery Contactor States
%         K1 = 0; K2 = 0; K3 = 0; K4 = 0;
% 
%         if Prchrgpnltytimer > 0
%             Prchrgpnltytimer = Prchrgpnltytimer - 1;
%         else
%             % Cooldown finished → check if PRECHARGE INHIBIT conditions still exist
%             if (Prchrgpnltytimer > Ke_t_PrechargeFailMaxPenalty) % Include the here || (HVBatPrechargeTemp > 60)
%                 % Inhibit condition persists → apply long penalty
%                 Prchrgpnltytimer = Ke_t_BPCM_Precharge_Fail_Penalty_Time;
%                 HVBatCntctrStat_Aux = 5;
%                 HVBatPrechgInbt = 1;
%             else
%                 % PRECHARGE INHIBIT conditions cleared → ready for retry
%                 Prchrgpnltytimer = 0;
%                 HVBatPrechgInbt = 0;
%                 HVBatCntctrStat_Aux = 0;
%             end
%         end
% 
%     case 6  % CONTACTOR CONTROL SHORTED STATE
%         % Set the Battery Contactor States
%         % K1 = 1; K2 = 0; K3 = 0; K4 = 0;
% 
% 
%     otherwise
%         K1 = 0; K2 = 0; K3 = 0; K4 = 0;
%         HVBatCntctrStat_Aux = 0;
% end
% 
% % --- Final Outputs ---
% HVBatCntctrStat = HVBatCntctrStat_Aux;
% Ke_t_HighVoltageBusActualPrechargeTime = max(0, VbusTargetHitIdx + ...
%     Min_Samples * (VbusTargetHitIdx ~= Unset_VbusTargetHitIdx));
% last_PrechargeAllw = PrechargeAllw;
% 
% end
